simulink model "TestTurbine_org"  (Simulink 10.0)
settings: Solver=ode45  StartTime=0.0  StopTime=10.0  RelTol=1e-3  EnableMultiTasking=on
libraries: Lib_TurboC_FlowStart_TMATSC x3, Lib_TurboC_Turbine_TMATSC x1
settings Model: Creator=tlavelle  LastModifiedBy=bhisma
settings DataIOCC: LimitDataPoints=on
settings OptimizationCC: ExpressionDepthLimit=2147483647
settings DebuggingCC: SolverPrmCheckMsg=warning  StateNameClashWarn=warning
settings GRTTargetCC: GeneratePreprocessorConditionals=Disable all  CombineOutputUpdateFcns=on  GRTInterface=off
settings ConfigComp: CovExternalEMLEnable=off

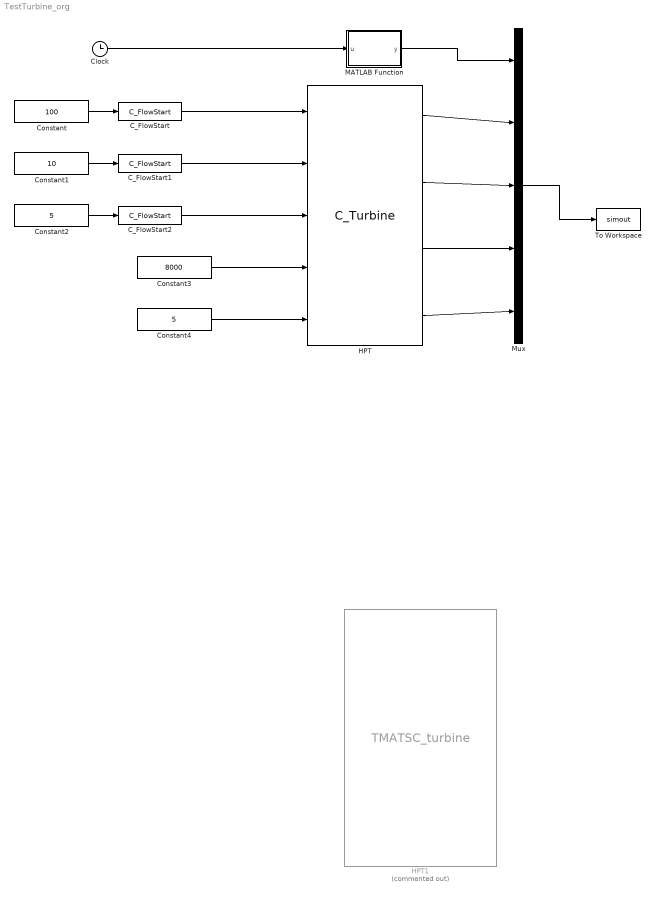
== system TestTurbine_org ==
  C_FlowStart : Lib_TurboC_FlowStart_TMATSC/C_FlowStart  Tt_M=2500  Pt_M=297.127  comp1_M=1  comp2_M=0  comp3_M=.025  comp4_M=0  comp5_M=0  comp6_M=0
  C_FlowStart1 : Lib_TurboC_FlowStart_TMATSC/C_FlowStart  Tt_M=1398  Pt_M=297.127  comp1_M=1  comp2_M=0  comp3_M=0  comp4_M=0  comp5_M=0  comp6_M=0
  C_FlowStart2 : Lib_TurboC_FlowStart_TMATSC/C_FlowStart  Tt_M=1398  Pt_M=297.127  comp1_M=1  comp2_M=0  comp3_M=0  comp4_M=0  comp5_M=0  comp6_M=0
  Clock : Clock
  Constant : Constant  Value=100
  Constant1 : Constant  Value=10
  Constant2 : Constant  Value=5
  Constant3 : Constant  Value=8000
  Constant4 : Constant  Value=5
  HPT : Lib_TurboC_Turbine_TMATSC/C_Turbine  MapFile_M='HPT1.map'  s_C_Nc_M=0.60  s_Wc_M=0.61  s_PR_M=0.95  s_eff_M=0.95  BSW1_M=1  BSW2_M=0  IDes_M=2  Ndes_M=7499  PRmapDes_M=4.9299  effDes_M=.913  NcDes_M=100
  HPT1 : M-S-Function  Commented=on  FunctionName=TMATSC_turbine  Parameters=MapFile_M ,NcDes_M ,effDes_M ,PRmapDes_M ,Ndes_M ,BSW1_M ,BSW2_M ,s_eff_M ,s_Wc_M ,s_C_Nc_M ,s_PR_M ,IDes_M  mask(T-MATS: Turbine Library Block, cantera){MapFile_M='HPT1.map', s_C_Nc_M=0.60, s_Wc_M=0.61, s_PR_M=0.95, s_eff_M=0.95, BSW1_M=1, BSW2_M=0, IDes_M=2, Ndes_M=7499, PRmapDes_M=4.9299, effDes_M=.913, NcDes_M=100}
      mask prompts: MapFile_M "Map File_M - Map File"; s_C_Nc_M "s_C_Nc_M - Input map speed scalar"; s_Wc_M "s_Wc_M - Input map correct weight flow scala"; s_PR_M "s_PR_M - Input map pressure ratio scalar"; s_eff_M "s_eff_M - Input map efficiency scalar"; BSW1_M "BSW1_M - Bleed 1 Switch (1 front 0 back)"; BSW2_M "BSW2_M - Bleed 2 Swtich (1 front 0 back )"; IDes_M "IDes_M - IDes"; Ndes_M "Ndes_M - N des"; PRmapDes_M "PRmapDes_M - Design Pressure Ratio Map"; effDes_M "effDes_M - Design efficiency"; NcDes_M "NcDes_M - Design Speed"
      mask help:
      | This block simulates the performance of a turbine using basic thermodynamic equations, properties, and table lookups.
      | This block makes use of the Cantera software package.
      mask Display:
      | color('blue'); port_label('input',1,'Flow In')
      | color('blue'); port_label('input',2,'Bleed 1')
      | color('blue'); port_label('input',3,'Bleed 2')
      | color('red'); port_label('input',4,'Speed')
      | color('green'); port_label('input',5,'PR')
      | 
      | color('blue'); port_label('output',1,'Flow Out')
      | color('green'); port_label('output',2,'Flow Error')
      | color('black'); port_label('output',3,'Power')
      | color('black'); port_label('output',4,'T_Data')
  MATLAB Function : MATLAB Function  TreatAsAtomicUnit=on
  Mux : Mux  Inputs=5
  To Workspace : ToWorkspace  VariableName=simout  SaveFormat=Timeseries  SampleTime=-1
  wires:
  Constant2/1 -> C_FlowStart2/1
  Constant1/1 -> C_FlowStart1/1
  Constant/1 -> C_FlowStart/1
  C_FlowStart/1 -> HPT/1
  C_FlowStart1/1 -> HPT/2
  C_FlowStart2/1 -> HPT/3
  Constant3/1 -> HPT/4
  Constant4/1 -> HPT/5
  Mux/1 -> To Workspace/1
  Clock/1 -> MATLAB Function/1(u)
  MATLAB Function/1(y) -> Mux/1
  HPT/1 -> Mux/2
  HPT/2 -> Mux/3
  HPT/3 -> Mux/4
  HPT/4 -> Mux/5

== matlab function MATLAB Function ==
  data: u input double; y output double
function y = fcn(u)
%#codegen
eml.extrinsic('set_param');
if u < 3
   set_param('TestTurbine/HPT','IDes_M','0');
elseif u< 6 
   set_param('TestTurbine/HPT','IDes_M','1'); 
else 
   set_param('TestTurbine/HPT','IDes_M','2'); 
end    
y = u;
